simulink model "Excavator_Control"  (R2024b)
settings: Solver=FixedStepAuto  StartTime=0.0  StopTime=10  FixedStep=0.01  RelTol=1e-3
libraries: simulink x1
settings Model: Creator=Amin  LastModifiedBy=galax
settings SolverCC: AlgebraicLoopSolver=TrustRegion
settings DataIOCC: ReturnWorkspaceOutputs=off
settings DebuggingCC: UnconnectedInputMsg=warning  UnconnectedOutputMsg=warning  UnconnectedLineMsg=warning  ArithmeticOperatorsInVariantConditions=warning
settings ModelReferenceCC: EnableRefExpFcnMdlSchedulingChecks=on
settings SFSimCC: SimUseLocalCustomCode=off  CustomCodeUndefinedFunction=UseInterfaceOnly
settings RTWCC: RTWUseLocalCustomCode=off  GPUComputeCapability=3.5

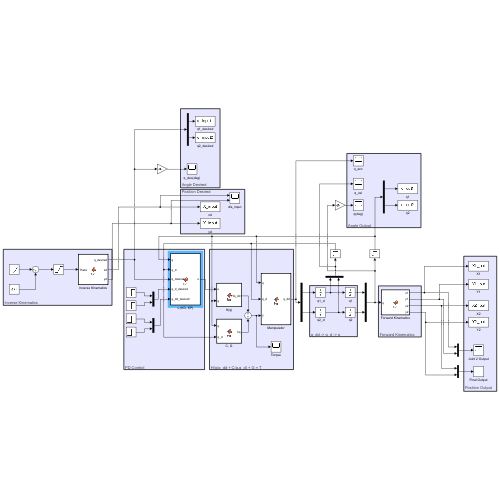
[thumbnail: Simulink's stored preview of the top-level diagram]
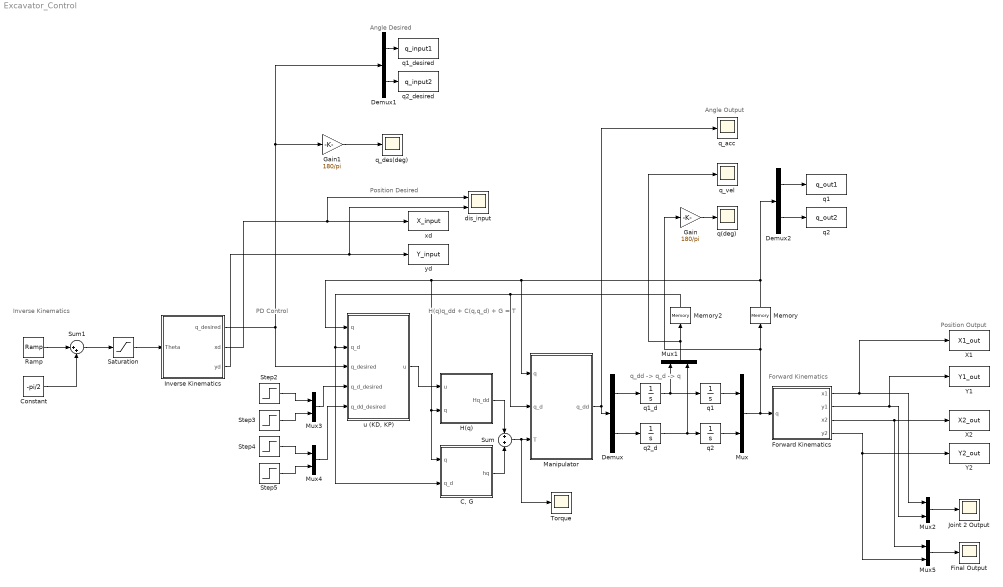
== system Excavator_Control ==
  note: Position Desired
  note: Position Output
  note: Angle Desired
  note: Angle Output
  note: q_dd -> q_d -> q
  note: Forward Kinematics
  note: PD Control
  note: H(q)q_dd + C(q,q_d) + G = T
  note: Inverse Kinematics
  " q1" : Integrator
  " q1_d" : Integrator
  " q2" : Integrator
  " q2_d" : Integrator
  "C, G" : MATLAB Function  TreatAsAtomicUnit=on
  Constant : Constant  Value=-pi/2
  Demux : Demux  Outputs=2
  Demux1 : Demux  Outputs=2
  Demux2 : Demux  Outputs=2
  Final Output : Scope
  Forward Kinematics : MATLAB Function  TreatAsAtomicUnit=on
  Gain : Gain  Gain=180/pi
  Gain1 : Gain  Gain=180/pi
  H(q) : MATLAB Function  TreatAsAtomicUnit=on
  Inverse Kinematics : MATLAB Function  TreatAsAtomicUnit=on
  Joint 2 Output : Scope
  Manipulator : MATLAB Function  TreatAsAtomicUnit=on
  Memory : Memory  InitialCondition=[0 0]
  Memory2 : Memory  InitialCondition=[0 0]
  Mux{,1..5} (6 alike) : Mux  Inputs=2
  Ramp : simulink/Sources/Ramp  slope=1  start=3  InitialOutput=0
  Saturation : Saturate  UpperLimit=pi/2  LowerLimit=-pi/2
  Step2 : Step  Before=0.01  After=0.01  SampleTime=0
  Step3 : Step  Before=0.01  After=0.01  SampleTime=0
  Step4 : Step  Before=0.001  After=0.001  SampleTime=0
  Step5 : Step  Before=0.001  After=0.001  SampleTime=0
  Sum : Sum  Inputs=+|+
  Sum1 : Sum  Inputs=|++
  Torque : Scope
  X1 : ToWorkspace  VariableName=X1_out  SaveFormat=Structure With Time  SampleTime=-1
  X2 : ToWorkspace  VariableName=X2_out  SaveFormat=Structure With Time  SampleTime=-1
  Y1 : ToWorkspace  VariableName=Y1_out  SaveFormat=Structure With Time  SampleTime=-1
  Y2 : ToWorkspace  VariableName=Y2_out  SaveFormat=Structure With Time  SampleTime=-1
  dis_input : Scope  NumInputPorts=2
  q(deg) : Scope
  q1 : ToWorkspace  VariableName=q_out1  SaveFormat=Structure With Time  SampleTime=-1
  q1_desired : ToWorkspace  VariableName=q_input1  SaveFormat=Structure With Time  SampleTime=-1
  q2 : ToWorkspace  VariableName=q_out2  SaveFormat=Structure With Time  SampleTime=-1
  q2_desired : ToWorkspace  VariableName=q_input2  SaveFormat=Structure With Time  SampleTime=-1
  q_acc : Scope
  q_des(deg) : Scope
  q_vel : Scope
  "u (KD, KP)" : MATLAB Function  TreatAsAtomicUnit=on
  xd : ToWorkspace  VariableName=X_input  SaveFormat=Structure With Time  SampleTime=-1
  yd : ToWorkspace  VariableName=Y_input  SaveFormat=Structure With Time  SampleTime=-1
  wires:
  " q1_d"/1 -> " q1"/1, Mux1/1
  " q2_d"/1 -> " q2"/1, Mux1/2
  Demux/1 -> " q1_d"/1
  Demux/2 -> " q2_d"/1
  " q2"/1 -> Mux/2
  Mux/1 -> Gain/1, Memory/1, Forward Kinematics/1(q)
  Mux1/1 -> Memory2/1, q_vel/1
  H(q)/1(Hq_dd) -> Sum/1
  "C, G"/1(hq) -> Sum/2
  Memory2/1 -> "C, G"/2(q_d), "u (KD, KP)"/2(q_d), Manipulator/2(q_d)
  Memory/1 -> Demux2/1, "u (KD, KP)"/1(q), "C, G"/1(q), H(q)/2(q), Manipulator/1(q)
  "u (KD, KP)"/1(u) -> H(q)/1(u)
  Forward Kinematics/1(x1) -> Mux2/1, X1/1
  Forward Kinematics/2(y1) -> Mux2/2, Y1/1
  Forward Kinematics/3(x2) -> X2/1, Mux5/1
  Forward Kinematics/4(y2) -> Y2/1, Mux5/2
  Step3/1 -> Mux3/2
  Step2/1 -> Mux3/1
  Step4/1 -> Mux4/1
  Step5/1 -> Mux4/2
  Mux4/1 -> "u (KD, KP)"/5(q_dd_desired)
  Inverse Kinematics/1(q_desired) -> Gain1/1, Demux1/1, "u (KD, KP)"/3(q_desired)
  Inverse Kinematics/2(xd) -> xd/1, dis_input/1
  Inverse Kinematics/3(yd) -> dis_input/2, yd/1
  Demux1/1 -> q1_desired/1
  Demux1/2 -> q2_desired/1
  Demux2/1 -> q1/1
  Demux2/2 -> q2/1
  Mux3/1 -> "u (KD, KP)"/4(q_d_desired)
  " q1"/1 -> Mux/1
  Manipulator/1(q_dd) -> q_acc/1, Demux/1
  Sum/1 -> Torque/1, Manipulator/3(T)
  Mux2/1 -> Joint 2 Output/1
  Mux5/1 -> Final Output/1
  Gain/1 -> q(deg)/1
  Gain1/1 -> q_des(deg)/1
  Sum1/1 -> Saturation/1
  Saturation/1 -> Inverse Kinematics/1(Theta)
  Constant/1 -> Sum1/2
  Ramp/1 -> Sum1/1

== matlab function Excavator_Control/H(q) ==
  data: u input; Hq_dd output; q input
%% Inertia Matrix
function Hq_dd = fcn(u, q)
l1 = 4.4; l2 = 2.2;
m1 = 1500; m2 = 700;
g = 9.81;

H11 = (1/3)*m1*(l1^2)+(1/3)*m2*(l2^2)+m2*(l1^2)+m2*l2*l2*cos(q(2));
H22 = (1/3)*m2*(l2^2)+(1/2)*m2*l1*l2*cos(q(2));
H12 = (1/3)*m2*(l2^2)+(1/2)*m2*l1*l2*cos(q(2));
H21 = (1/3)*m2*(l2^2);

H = [H11 H12; H21 H22];

% Inertia Term
Hq_dd = H*u;

== matlab function Excavator_Control/Manipulator ==
  data: q input; q_dd output; q_d input; T input
%% H(q)q_dd + C(q,q_d) + G = T
function q_dd = fcn(q, q_d, T)
l1 = 4.4; l2 = 2.2;
m1 = 1500; m2 = 700;
g = 9.81;

H11 = (1/3)*m1*(l1^2)+(1/3)*m2*(l2^2)+m2*(l1^2)+m2*l2*l2*cos(q(2));
H22 = (1/3)*m2*(l2^2)+(1/2)*m2*l1*l2*cos(q(2));
H12 = (1/3)*m2*(l2^2)+(1/2)*m2*l1*l2*cos(q(2));
H21 = (1/3)*m2*(l2^2);

H = [H11 H12; H21 H22];

h1 = - m2*l1*l2*sin(q(2))*q_d(1)*q_d(2) - (1/2)*m2*l1*l2*sin(q(2))*(q_d(2)^2);
h2 = (1/2)*m2*l2*l2*sin(q(2))*(q_d(1)^2);

C = [h1; h2];

g1 = (1/2)*m1*l1*g*cos(q(1)) + (1/2)*m2*l2*g*cos(q(1)+q(2)) + m2*l1*g*cos(q(1));
g2 = (1/2)*m2*l2*g*cos(q(1)+q(2));

G = [g1; g2];

%% Angular Accerlation
q_dd = H \ (T - C - G);

== matlab function Excavator_Control/C, G ==
  data: q input; hq output; q_d input
%% Coriolis and Centrifugal Force Matrices / Gravity Vector
function hq = fcn(q, q_d)
l1 = 4.4; l2 = 2.2;
m1 = 1500; m2 = 700;
g = 9.81;

h1 = - m2*l1*l2*sin(q(2))*q_d(1)*q_d(2) - (1/2)*m2*l1*l2*sin(q(2))*(q_d(2)^2);
h2 = (1/2)*m2*l2*l2*sin(q(2))*(q_d(1)^2);

C = [h1; h2];

g1 = (1/2)*m1*l1*g*cos(q(1)) + (1/2)*m2*l2*g*cos(q(1)+q(2)) + m2*l1*g*cos(q(1));
g2 = (1/2)*m2*l2*g*cos(q(1)+q(2));

G = [g1; g2];

% Coriolis and Centrifugal Term + Gravity Term
hq = C + G;

== matlab function Excavator_Control/Forward Kinematics ==
  data: q input; x1 output; y1 output; x2 output; y2 output
%% Forward Kinematics
function [x1,y1,x2,y2] = fcn(q)
l1 = 4.4; l2 = 2.2;
g = 9.81;

% Joint 2 location
x1 = l1*cos(q(1));
y1 = l1*sin(q(1));

% Final location
x2 = l1*cos(q(1))+l2*cos(q(1)+q(2));
y2 = l1*sin(q(1))+l2*sin(q(1)+q(2));

== matlab function Excavator_Control/u (KD, KP) ==
  data: q input; u output; q_d input; q_desired input; q_d_desired input; q_dd_desired input
    %% PD Control
function u = fcn(q, q_d, q_desired, q_d_desired, q_dd_desired)
KD = 40;
KP = 200;

q_tilted = q - q_desired;
q_d_tilted = q_d - q_d_desired;

u = q_dd_desired-(KD*(q_d_tilted))-(KP*(q_tilted));

== matlab function Excavator_Control/Inverse Kinematics ==
  data: q_desired output; Theta input; xd output; yd output
function [q_desired, xd, yd] = fcn(Theta)
%% Parameters
l1 = 4.4; l2 = 2.2;
x0 = 0; y0 = 0;
r = 5.5;

%% Trajectory Design (Circle)
xd = x0 + r*cos(Theta); 
yd = y0 + r*sin(Theta);

%% Inverse Kinematic
C = (xd^2 + yd^2 - l1^2 - l2^2) / (2 * l1 * l2);
D = - sqrt(1 - C^2);
q2_desired = atan2(D, C);

q1_part1 = atan2(yd, xd);
q1_part2 = atan2(l2*sin(q2_desired), l1+l2*cos(q2_desired));
q1_desired = q1_part1 - q1_part2;

% Output Theta
q_desired = [q1_desired; q2_desired];
